simulink model "TrafficLed_Stateflow_App"  (R2024a)
settings: Solver=VariableStepAuto  StartTime=0.0  StopTime=1000  RelTol=1e-3
settings Model: Creator=DELL  LastModifiedBy=DELL

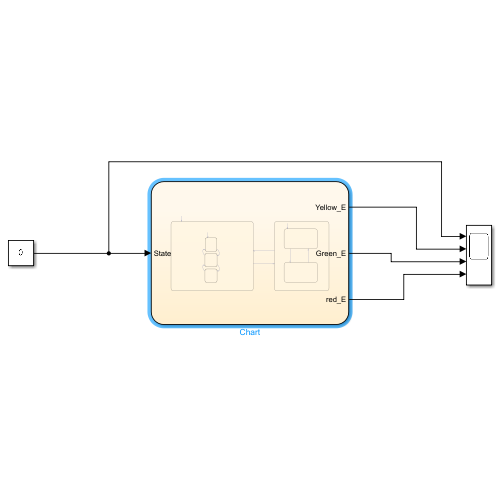
[thumbnail: Simulink's stored preview of the top-level diagram]
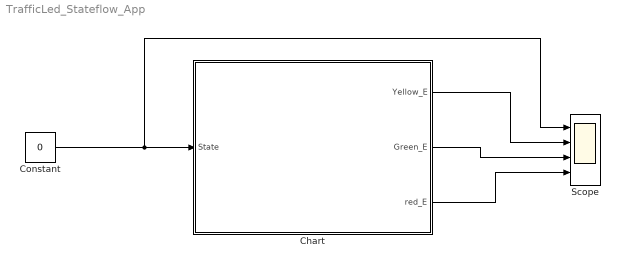
== system TrafficLed_Stateflow_App ==
  Chart : Stateflow chart  TreatAsAtomicUnit=on
  Constant : Constant  Value=0
  Scope : Scope  NumInputPorts=4
  wires:
  Chart/1(Yellow_E) -> Scope/2
  Chart/2(Green_E) -> Scope/3
  Chart/3(red_E) -> Scope/4
  Constant/1 -> Scope/1, Chart/1(State)

== stateflow chart TrafficLed_Stateflow_App/Chart ==
  state Normal_S
    state StopS
      en:
      red_E=1;
      Yellow_E=0;
      Green_E=0;
    state ReadyS
      en:
      Yellow_E=1;
      red_E=0;
      Green_E=0;
    state GoS
      en:
      Green_E=1;
      red_E=0;
      Yellow_E=0;
    (default) -> StopS
    ReadyS -> StopS [order 1] : after(5,sec)
    StopS -> ReadyS : after(120,sec)
    GoS -> ReadyS : after(40,sec)
    ReadyS -> GoS [order 2] : after(5,sec)
  state Fault_S
    state LedON
      en:
      red_E=1;
    state LedOff
      en:
      red_E=0;
    (default) -> LedON
    LedON -> LedOff : after(1,msec)
    LedOff -> LedON : after(1,msec)
  (default) -> Normal_S
  Fault_S -> Normal_S : [State==0]
  Normal_S -> Fault_S : [State==1]
  data: State input; Yellow_E output; Green_E output; red_E output
